simulink model "bitsel"  (Simulink 6.2)
settings: Solver=ode45  StartTime=0.0  StopTime=10.0  RelTol=1e-3
libraries: xbsIndex_r3 x74
settings Model: LastModifiedBy=mdexter
settings DebuggingCC: SolverPrmCheckMsg=warning

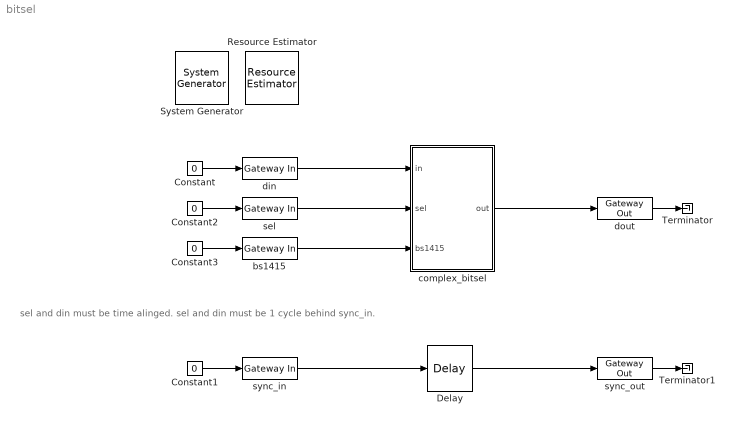
== system bitsel ==
  note: sel and din must be time alinged.
      | sel and din must be 1 cycle behind sync_in.
  " System Generator" : xbsIndex_r3/ System Generator  Tag=genX  xilinxfamily=Virtex2P  part=xc2vp40  speed=-6  package=ff1152  synthesis_tool=XST  directory=./bitsel_core  testbench=off  simulink_period=1  sysclk_period=100  incr_netlist=off  trim_vbits=Everywhere in SubSystem  dbl_ovrd=According to Block Masks  core_generation=According to Block Masks  run_coregen=off  deprecated_control=off  eval_field=0
      settings: AttributesFormatString=System\nGenerator
  Constant{,1..3} (4 alike) : Constant  Value=0
  Delay : xbsIndex_r3/Delay  latency=2  reg_retiming=off  explicit_period=off  period=1  en=off  accept_only_valid=off  init_zero=on  dbl_ovrd=off  show_param=off
      settings: xl_area=[1 1 0 1 0 0 0]
  Resource Estimator : xbsIndex_r3/Resource Estimator  Tag=resEstTag  xl_estimator_area=[342 135 0 641 52 0 0]  xl_use_estimator_area=off  simulink_period=1  mrp_directory=./bitsel_core
      settings: AttributesFormatString=Resource\nEstimator
  Terminator : Terminator
  Terminator1 : Terminator
  bs1415 : xbsIndex_r3/Gateway In  arith_type=Unsigned  n_bits=16  bin_pt=0  quantization=Truncate  overflow=Wrap  period=1  timing_constraint=None  locs_specified=off  LOCs={}  needs_fixed_name=off  dbl_ovrd=off  show_param=off
      settings: xl_area=[0 0 0 0 4 0 0]
  complex_bitsel : Subsystem
      settings: AttributesFormatString=latency = 2
  din : xbsIndex_r3/Gateway In  arith_type=Unsigned  n_bits=38  bin_pt=0  quantization=Truncate  overflow=Wrap  period=1  timing_constraint=None  locs_specified=off  LOCs={}  needs_fixed_name=off  dbl_ovrd=off  show_param=off
      settings: xl_area=[0 0 0 0 38 0 0]
  dout : xbsIndex_r3/Gateway Out  output_type=Double  nbits=8  bin_pt=6  arith_type=Boolean  quantization=Truncate  overflow=Wrap  hdl_port=on  timing_constraint=None  locs_specified=off  LOCs={}  needs_fixed_name=off  show_param=off
      settings: xl_area=[0 0 0 0 8 0 0]
  sel : xbsIndex_r3/Gateway In  arith_type=Unsigned  n_bits=4  bin_pt=0  quantization=Truncate  overflow=Wrap  period=1  timing_constraint=None  locs_specified=off  LOCs={}  needs_fixed_name=off  dbl_ovrd=off  show_param=off
      settings: xl_area=[0 0 0 0 4 0 0]
  sync_in : xbsIndex_r3/Gateway In  arith_type=Boolean  n_bits=36  bin_pt=0  quantization=Truncate  overflow=Wrap  period=1  timing_constraint=None  locs_specified=off  LOCs={}  needs_fixed_name=off  dbl_ovrd=off  show_param=off
      settings: xl_area=[0 0 0 0 1 0 0]
  sync_out : xbsIndex_r3/Gateway Out  output_type=Double  nbits=8  bin_pt=6  arith_type=Boolean  quantization=Truncate  overflow=Wrap  hdl_port=on  timing_constraint=None  locs_specified=off  LOCs={}  needs_fixed_name=off  show_param=off
      settings: xl_area=[0 0 0 0 1 0 0]
  wires:
  Constant/1 -> din/1
  Constant2/1 -> sel/1
  dout/1 -> Terminator/1
  Constant1/1 -> sync_in/1
  sync_out/1 -> Terminator1/1
  sync_in/1 -> Delay/1
  Delay/1 -> sync_out/1
  din/1 -> complex_bitsel/1(in)
  sel/1 -> complex_bitsel/2(sel)
  complex_bitsel/1(out) -> dout/1
  Constant3/1 -> bs1415/1
  bs1415/1 -> complex_bitsel/3(bs1415)

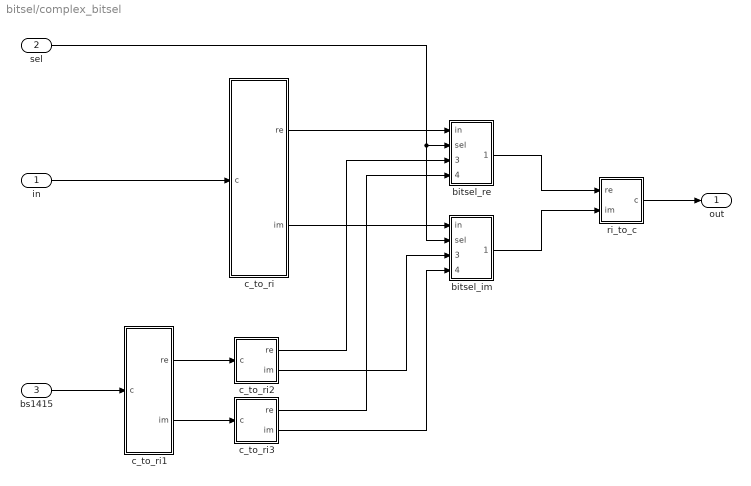
== system bitsel/complex_bitsel ==
  in : Inport  Port=1  LatchInput=off
  sel : Inport  Port=2  LatchInput=off
  bs1415 : Inport  Port=3  LatchInput=off
  bitsel_im : Subsystem
      settings: AttributesFormatString=latency = 2
  bitsel_re : Subsystem
      settings: AttributesFormatString=latency = 2
  c_to_ri : Subsystem  mask(Complex to Real-Imag){n_bits=19, bin_pt=0}
      mask prompts: n_bits "Bit Width"; bin_pt "Binary Point"
      mask help: Outputs real and imaginary components of a complex input.
      mask init:
      | c_to_ri_init(gcb,n_bits,bin_pt);
      settings: AttributesFormatString=19_0 r/i
      mask Help:
      | <pre>
      | Description::
      | 
      | Outputs real and imaginary components of a complex input.
      | Useful for simplifying interconnects.
      | See also: Real-Imag to Complex (ri_to_c)
      | 
      | Mask Parameters::
      | 
      | Bit Width (n_bits): Specifies the width of the real/imaginary components.
      | Assumed equal for both components.
      | 
      | Binary Point (bin_pt): Specifies the binary point location in the real/imaginary components.
      | Assumed equal for both components.
      | </pre>
  c_to_ri1 : Subsystem  mask(Complex to Real-Imag){n_bits=8, bin_pt=0}
      mask prompts: n_bits "Bit Width"; bin_pt "Binary Point"
      mask help: Outputs real and imaginary components of a complex input.
      mask init:
      | c_to_ri_init(gcb,n_bits,bin_pt);
      settings: AttributesFormatString=8_0 r/i
      mask Help:
      | <pre>
      | Description::
      | 
      | Outputs real and imaginary components of a complex input.
      | Useful for simplifying interconnects.
      | See also: Real-Imag to Complex (ri_to_c)
      | 
      | Mask Parameters::
      | 
      | Bit Width (n_bits): Specifies the width of the real/imaginary components.
      | Assumed equal for both components.
      | 
      | Binary Point (bin_pt): Specifies the binary point location in the real/imaginary components.
      | Assumed equal for both components.
      | </pre>
  c_to_ri2 : Subsystem  mask(Complex to Real-Imag){n_bits=4, bin_pt=0}
      mask prompts: n_bits "Bit Width"; bin_pt "Binary Point"
      mask help: Outputs real and imaginary components of a complex input.
      mask init:
      | c_to_ri_init(gcb,n_bits,bin_pt);
      settings: AttributesFormatString=4_0 r/i
      mask Help:
      | <pre>
      | Description::
      | 
      | Outputs real and imaginary components of a complex input.
      | Useful for simplifying interconnects.
      | See also: Real-Imag to Complex (ri_to_c)
      | 
      | Mask Parameters::
      | 
      | Bit Width (n_bits): Specifies the width of the real/imaginary components.
      | Assumed equal for both components.
      | 
      | Binary Point (bin_pt): Specifies the binary point location in the real/imaginary components.
      | Assumed equal for both components.
      | </pre>
  c_to_ri3 : Subsystem  mask(Complex to Real-Imag){n_bits=4, bin_pt=0}
      mask prompts: n_bits "Bit Width"; bin_pt "Binary Point"
      mask help: Outputs real and imaginary components of a complex input.
      mask init:
      | c_to_ri_init(gcb,n_bits,bin_pt);
      settings: AttributesFormatString=4_0 r/i
      mask Help:
      | <pre>
      | Description::
      | 
      | Outputs real and imaginary components of a complex input.
      | Useful for simplifying interconnects.
      | See also: Real-Imag to Complex (ri_to_c)
      | 
      | Mask Parameters::
      | 
      | Bit Width (n_bits): Specifies the width of the real/imaginary components.
      | Assumed equal for both components.
      | 
      | Binary Point (bin_pt): Specifies the binary point location in the real/imaginary components.
      | Assumed equal for both components.
      | </pre>
  ri_to_c : Subsystem  mask(Real-Imag to Complex){}
      mask help: Concatenates real and imaginary inputs into a complex output.
      mask init:
      | ri_to_c_init(gcb);
      mask Help:
      | <pre>
      | Description::
      | 
      | Concatenates a real and imaginary input into a complex output.
      | Useful for simplifying interconnects.
      | See also: Complex to Real-Imag (c_to_ri)
      | 
      | Mask Parameters::
      | 
      | (N/A)
      | </pre>
  out : Outport
  wires:
  in/1 -> c_to_ri/1(c)
  sel/1 -> bitsel_im/2(sel), bitsel_re/2(sel)
  c_to_ri/1(re) -> bitsel_re/1(in)
  c_to_ri/2(im) -> bitsel_im/1(in)
  bitsel_re/1(out) -> ri_to_c/1(re)
  ri_to_c/1(c) -> out/1
  bitsel_im/1(out) -> ri_to_c/2(im)
  c_to_ri1/1(re) -> c_to_ri2/1(c)
  c_to_ri1/2(im) -> c_to_ri3/1(c)
  c_to_ri2/1(re) -> bitsel_re/3(bs14)
  c_to_ri3/1(re) -> bitsel_re/4(bs15)
  c_to_ri2/2(im) -> bitsel_im/3(bs14)
  c_to_ri3/2(im) -> bitsel_im/4(bs15)
  bs1415/1 -> c_to_ri1/1(c)

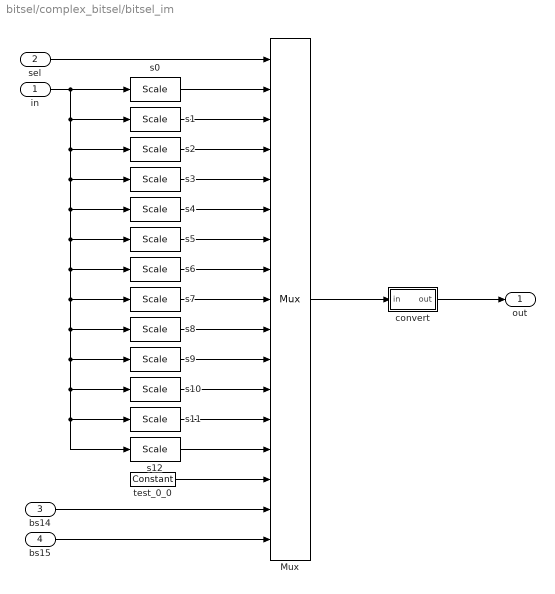
== system bitsel/complex_bitsel/bitsel_im ==
  in : Inport  Port=1  LatchInput=off
  sel : Inport  Port=2  LatchInput=off
  bs14 : Inport  Port=3  LatchInput=off
  bs15 : Inport  Port=4  LatchInput=off
  Mux : xbsIndex_r3/Mux  inputs=16  precision=Full  arith_type="Signed  (2's comp)"  n_bits=8  bin_pt=2  quantization=Truncate  overflow=Wrap  latency=1  explicit_period=off  period=1  en=off  dbl_ovrd=off  show_param=on  mux_type=off  use_rpm=on  gen_core=off
      settings: xl_area=[140 31 0 279 0 0 0]
  convert : Subsystem  mask(Convert (cast)){bin_pt_in=15, n_bits_out=4, bin_pt_out=0, quantization=Round  (unbiased: Even Values), overflow=Saturate, latency=1}
      mask prompts: bin_pt_in "Binary Point In"; n_bits_out "Bit Width Out"; bin_pt_out "Binary Point Out"
      mask help: Convert input value to the specified bit width and precision.
      mask init:
      | convert_init(gcb, ...
      |     bin_pt_in, ...
      |     n_bits_out,bin_pt_out, ...
      |     quantization,overflow,latency);
      settings: AttributesFormatString=|
      | N_15 ==> 4_0
      | round even, saturate
      | latency = 1
      mask Help:
      | <pre>
      | Description::
      | 
      | Outputs converted version of the input.
      | 
      | Mask Parameters::
      | 
      | Binary Point In (bin_pt_in): Specifies the binary point location in the input.
      | 
      | Bit Width Out (n_bits_out): Specifies the width of the output.
      | 
      | Binary Point Out (bin_pt_out): Specifies the binary point location in the output.
      | 
      | Quantization (quantization): Specifies quantization handling.
      | 
      | Overflow (overflow): Specifies overflow handling.
      | 
      | Latency (latency): Specifies the latency of the underlying adder block, which is the overall
      | latency of this block as well.
      | </pre>
      mask StyleString: edit,edit,edit,popup(Truncate|Round  (unbiased: +/- Inf)|Round  (unbiased: Even Values)|Round  (unbiased: Zero)|Round  (unbiased: Odd Values)|Round  (biased: Up)|Round  (biased: Down)),popup(Wrap|Saturate|Error),edit
  s0 : xbsIndex_r3/Scale  scale_factor=-15  explicit_period=off  period=1  dbl_ovrd=off
  s1 : xbsIndex_r3/Scale  scale_factor=-14  explicit_period=off  period=1  dbl_ovrd=off
  s10 : xbsIndex_r3/Scale  scale_factor=-5  explicit_period=off  period=1  dbl_ovrd=off
  s11 : xbsIndex_r3/Scale  scale_factor=-4  explicit_period=off  period=1  dbl_ovrd=off
  s12 : xbsIndex_r3/Scale  scale_factor=-3  explicit_period=off  period=1  dbl_ovrd=off
  s2 : xbsIndex_r3/Scale  scale_factor=-13  explicit_period=off  period=1  dbl_ovrd=off
  s3 : xbsIndex_r3/Scale  scale_factor=-12  explicit_period=off  period=1  dbl_ovrd=off
  s4 : xbsIndex_r3/Scale  scale_factor=-11  explicit_period=off  period=1  dbl_ovrd=off
  s5 : xbsIndex_r3/Scale  scale_factor=-10  explicit_period=off  period=1  dbl_ovrd=off
  s6 : xbsIndex_r3/Scale  scale_factor=-9  explicit_period=off  period=1  dbl_ovrd=off
  s7 : xbsIndex_r3/Scale  scale_factor=-8  explicit_period=off  period=1  dbl_ovrd=off
  s8 : xbsIndex_r3/Scale  scale_factor=-7  explicit_period=off  period=1  dbl_ovrd=off
  s9 : xbsIndex_r3/Scale  scale_factor=-6  explicit_period=off  period=1  dbl_ovrd=off
  test_0_0 : xbsIndex_r3/Constant  const=0  equ=P=C  arith_type="Signed  (2's comp)"  n_bits=4  bin_pt=0  opselect=C  inp2=PCIN>>17  opr=+  inp1=P  carry=CIN  iostate=0  explicit_period=on  period=1  dbl_ovrd=off
  out : Outport
  wires:
  in/1 -> s11/1, s12/1, s10/1, s9/1, s8/1, s7/1, s6/1, s5/1, s4/1, s3/1, s2/1, s1/1, s0/1
  s0/1 -> Mux/2
  s1/1 -> Mux/3
  s2/1 -> Mux/4
  s3/1 -> Mux/5
  s4/1 -> Mux/6
  s5/1 -> Mux/7
  s6/1 -> Mux/8
  s7/1 -> Mux/9
  s8/1 -> Mux/10
  s9/1 -> Mux/11
  s10/1 -> Mux/12
  s11/1 -> Mux/13
  s12/1 -> Mux/14
  test_0_0/1 -> Mux/15
  bs14/1 -> Mux/16
  bs15/1 -> Mux/17
  Mux/1 -> convert/1(in)
  sel/1 -> Mux/1
  convert/1(out) -> out/1

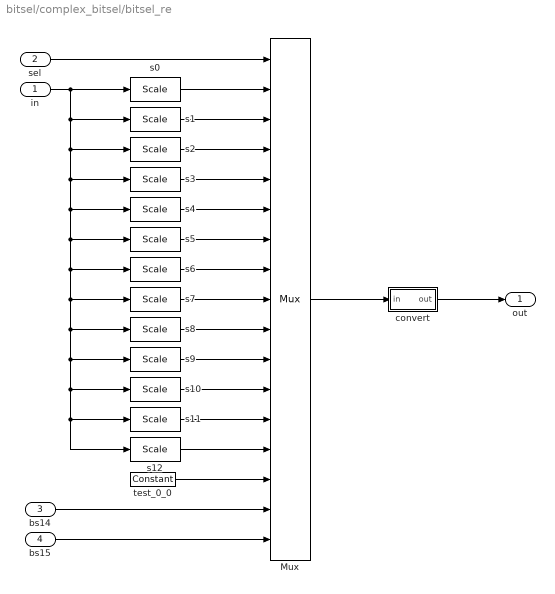
== system bitsel/complex_bitsel/bitsel_re ==
  in : Inport  Port=1  LatchInput=off
  sel : Inport  Port=2  LatchInput=off
  bs14 : Inport  Port=3  LatchInput=off
  bs15 : Inport  Port=4  LatchInput=off
  Mux : xbsIndex_r3/Mux  inputs=16  precision=Full  arith_type="Signed  (2's comp)"  n_bits=8  bin_pt=2  quantization=Truncate  overflow=Wrap  latency=1  explicit_period=off  period=1  en=off  dbl_ovrd=off  show_param=on  mux_type=off  use_rpm=on  gen_core=off
      settings: xl_area=[140 31 0 279 0 0 0]
  convert : Subsystem  mask(Convert (cast)){bin_pt_in=15, n_bits_out=4, bin_pt_out=0, quantization=Round  (unbiased: Even Values), overflow=Saturate, latency=1}
      mask prompts: bin_pt_in "Binary Point In"; n_bits_out "Bit Width Out"; bin_pt_out "Binary Point Out"
      mask help: Convert input value to the specified bit width and precision.
      mask init:
      | convert_init(gcb, ...
      |     bin_pt_in, ...
      |     n_bits_out,bin_pt_out, ...
      |     quantization,overflow,latency);
      settings: AttributesFormatString=|
      | N_15 ==> 4_0
      | round even, saturate
      | latency = 1
      mask Help:
      | <pre>
      | Description::
      | 
      | Outputs converted version of the input.
      | 
      | Mask Parameters::
      | 
      | Binary Point In (bin_pt_in): Specifies the binary point location in the input.
      | 
      | Bit Width Out (n_bits_out): Specifies the width of the output.
      | 
      | Binary Point Out (bin_pt_out): Specifies the binary point location in the output.
      | 
      | Quantization (quantization): Specifies quantization handling.
      | 
      | Overflow (overflow): Specifies overflow handling.
      | 
      | Latency (latency): Specifies the latency of the underlying adder block, which is the overall
      | latency of this block as well.
      | </pre>
      mask StyleString: edit,edit,edit,popup(Truncate|Round  (unbiased: +/- Inf)|Round  (unbiased: Even Values)|Round  (unbiased: Zero)|Round  (unbiased: Odd Values)|Round  (biased: Up)|Round  (biased: Down)),popup(Wrap|Saturate|Error),edit
  s0 : xbsIndex_r3/Scale  scale_factor=-15  explicit_period=off  period=1  dbl_ovrd=off
  s1 : xbsIndex_r3/Scale  scale_factor=-14  explicit_period=off  period=1  dbl_ovrd=off
  s10 : xbsIndex_r3/Scale  scale_factor=-5  explicit_period=off  period=1  dbl_ovrd=off
  s11 : xbsIndex_r3/Scale  scale_factor=-4  explicit_period=off  period=1  dbl_ovrd=off
  s12 : xbsIndex_r3/Scale  scale_factor=-3  explicit_period=off  period=1  dbl_ovrd=off
  s2 : xbsIndex_r3/Scale  scale_factor=-13  explicit_period=off  period=1  dbl_ovrd=off
  s3 : xbsIndex_r3/Scale  scale_factor=-12  explicit_period=off  period=1  dbl_ovrd=off
  s4 : xbsIndex_r3/Scale  scale_factor=-11  explicit_period=off  period=1  dbl_ovrd=off
  s5 : xbsIndex_r3/Scale  scale_factor=-10  explicit_period=off  period=1  dbl_ovrd=off
  s6 : xbsIndex_r3/Scale  scale_factor=-9  explicit_period=off  period=1  dbl_ovrd=off
  s7 : xbsIndex_r3/Scale  scale_factor=-8  explicit_period=off  period=1  dbl_ovrd=off
  s8 : xbsIndex_r3/Scale  scale_factor=-7  explicit_period=off  period=1  dbl_ovrd=off
  s9 : xbsIndex_r3/Scale  scale_factor=-6  explicit_period=off  period=1  dbl_ovrd=off
  test_0_0 : xbsIndex_r3/Constant  const=0  equ=P=C  arith_type="Signed  (2's comp)"  n_bits=4  bin_pt=0  opselect=C  inp2=PCIN>>17  opr=+  inp1=P  carry=CIN  iostate=0  explicit_period=on  period=1  dbl_ovrd=off
  out : Outport
  wires:
  in/1 -> s11/1, s12/1, s10/1, s9/1, s8/1, s7/1, s6/1, s5/1, s4/1, s3/1, s2/1, s1/1, s0/1
  s0/1 -> Mux/2
  s1/1 -> Mux/3
  s2/1 -> Mux/4
  s3/1 -> Mux/5
  s4/1 -> Mux/6
  s5/1 -> Mux/7
  s6/1 -> Mux/8
  s7/1 -> Mux/9
  s8/1 -> Mux/10
  s9/1 -> Mux/11
  s10/1 -> Mux/12
  s11/1 -> Mux/13
  s12/1 -> Mux/14
  test_0_0/1 -> Mux/15
  bs14/1 -> Mux/16
  bs15/1 -> Mux/17
  Mux/1 -> convert/1(in)
  sel/1 -> Mux/1
  convert/1(out) -> out/1

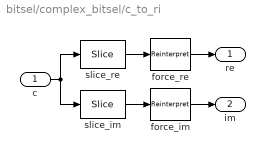
== system bitsel/complex_bitsel/c_to_ri ==
  c : Inport  Port=1  LatchInput=off
  force_im : xbsIndex_r3/Reinterpret  force_arith_type=on  arith_type="Signed  (2's comp)"  force_bin_pt=on  bin_pt=0  force_valid=on
  force_re : xbsIndex_r3/Reinterpret  force_arith_type=on  arith_type="Signed  (2's comp)"  force_bin_pt=on  bin_pt=0  force_valid=on
  slice_im : xbsIndex_r3/Slice  mode=Lower Bit Location + Width  nbits=19  bit1=0  base1=MSB of Input  bit0=0  base0=LSB of Input  boolean_output=off  explicit_period=off  period=1  dbl_ovrd=off
  slice_re : xbsIndex_r3/Slice  mode=Upper Bit Location + Width  nbits=19  bit1=0  base1=MSB of Input  bit0=0  base0=LSB of Input  boolean_output=off  explicit_period=off  period=1  dbl_ovrd=off
  re : Outport
  im : Outport  Port=2
  wires:
  slice_re/1 -> force_re/1
  slice_im/1 -> force_im/1
  force_re/1 -> re/1
  force_im/1 -> im/1
  c/1 -> slice_re/1, slice_im/1

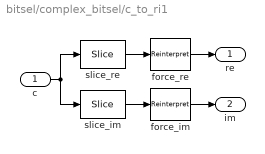
== system bitsel/complex_bitsel/c_to_ri1 ==
  c : Inport  Port=1  LatchInput=off
  force_im : xbsIndex_r3/Reinterpret  force_arith_type=on  arith_type="Signed  (2's comp)"  force_bin_pt=on  bin_pt=0  force_valid=on
  force_re : xbsIndex_r3/Reinterpret  force_arith_type=on  arith_type="Signed  (2's comp)"  force_bin_pt=on  bin_pt=0  force_valid=on
  slice_im : xbsIndex_r3/Slice  mode=Lower Bit Location + Width  nbits=8  bit1=0  base1=MSB of Input  bit0=0  base0=LSB of Input  boolean_output=off  explicit_period=off  period=1  dbl_ovrd=off
  slice_re : xbsIndex_r3/Slice  mode=Upper Bit Location + Width  nbits=8  bit1=0  base1=MSB of Input  bit0=0  base0=LSB of Input  boolean_output=off  explicit_period=off  period=1  dbl_ovrd=off
  re : Outport
  im : Outport  Port=2
  wires:
  slice_re/1 -> force_re/1
  slice_im/1 -> force_im/1
  force_re/1 -> re/1
  force_im/1 -> im/1
  c/1 -> slice_re/1, slice_im/1

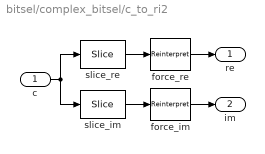
== system bitsel/complex_bitsel/c_to_ri2 ==
  c : Inport  Port=1  LatchInput=off
  force_im : xbsIndex_r3/Reinterpret  force_arith_type=on  arith_type="Signed  (2's comp)"  force_bin_pt=on  bin_pt=0  force_valid=on
  force_re : xbsIndex_r3/Reinterpret  force_arith_type=on  arith_type="Signed  (2's comp)"  force_bin_pt=on  bin_pt=0  force_valid=on
  slice_im : xbsIndex_r3/Slice  mode=Lower Bit Location + Width  nbits=4  bit1=0  base1=MSB of Input  bit0=0  base0=LSB of Input  boolean_output=off  explicit_period=off  period=1  dbl_ovrd=off
  slice_re : xbsIndex_r3/Slice  mode=Upper Bit Location + Width  nbits=4  bit1=0  base1=MSB of Input  bit0=0  base0=LSB of Input  boolean_output=off  explicit_period=off  period=1  dbl_ovrd=off
  re : Outport
  im : Outport  Port=2
  wires:
  slice_re/1 -> force_re/1
  slice_im/1 -> force_im/1
  force_re/1 -> re/1
  force_im/1 -> im/1
  c/1 -> slice_re/1, slice_im/1

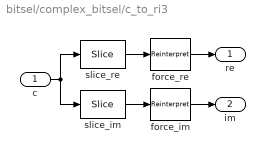
== system bitsel/complex_bitsel/c_to_ri3 ==
  c : Inport  Port=1  LatchInput=off
  force_im : xbsIndex_r3/Reinterpret  force_arith_type=on  arith_type="Signed  (2's comp)"  force_bin_pt=on  bin_pt=0  force_valid=on
  force_re : xbsIndex_r3/Reinterpret  force_arith_type=on  arith_type="Signed  (2's comp)"  force_bin_pt=on  bin_pt=0  force_valid=on
  slice_im : xbsIndex_r3/Slice  mode=Lower Bit Location + Width  nbits=4  bit1=0  base1=MSB of Input  bit0=0  base0=LSB of Input  boolean_output=off  explicit_period=off  period=1  dbl_ovrd=off
  slice_re : xbsIndex_r3/Slice  mode=Upper Bit Location + Width  nbits=4  bit1=0  base1=MSB of Input  bit0=0  base0=LSB of Input  boolean_output=off  explicit_period=off  period=1  dbl_ovrd=off
  re : Outport
  im : Outport  Port=2
  wires:
  slice_re/1 -> force_re/1
  slice_im/1 -> force_im/1
  force_re/1 -> re/1
  force_im/1 -> im/1
  c/1 -> slice_re/1, slice_im/1

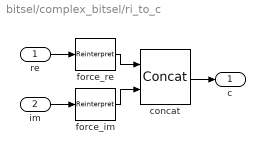
== system bitsel/complex_bitsel/ri_to_c ==
  re : Inport  Port=1  LatchInput=off
  im : Inport  Port=2  LatchInput=off
  concat : xbsIndex_r3/Concat  num_inputs=2  explicit_period=off  period=1  dbl_ovrd=off
  force_im : xbsIndex_r3/Reinterpret  force_arith_type=on  arith_type=Unsigned  force_bin_pt=on  bin_pt=0  force_valid=on
  force_re : xbsIndex_r3/Reinterpret  force_arith_type=on  arith_type=Unsigned  force_bin_pt=on  bin_pt=0  force_valid=on
  c : Outport
  wires:
  force_re/1 -> concat/1
  force_im/1 -> concat/2
  re/1 -> force_re/1
  concat/1 -> c/1
  im/1 -> force_im/1

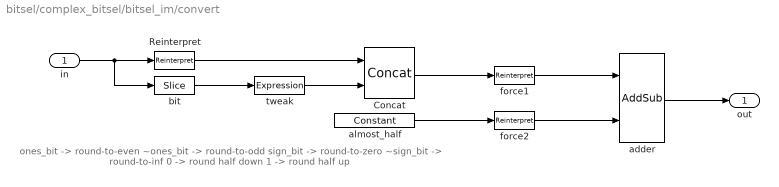
== system bitsel/complex_bitsel/bitsel_im/convert ==
  note: ones_bit -> round-to-even
      | ~ones_bit -> round-to-odd
      | sign_bit -> round-to-zero
      | ~sign_bit -> round-to-inf
      | 0 -> round half down
      | 1 -> round half up
  in : Inport  Port=1  LatchInput=off
  Concat : xbsIndex_r3/Concat  num_inputs=2  explicit_period=off  period=1  dbl_ovrd=off
  Reinterpret : xbsIndex_r3/Reinterpret  force_arith_type=on  arith_type=Unsigned  force_bin_pt=on  bin_pt=0  force_valid=on
  adder : xbsIndex_r3/AddSub  mode=Addition  precision=User Defined  arith_type="Signed  (2's comp)"  n_bits=4  bin_pt=0  quantization=Truncate  overflow=Saturate  latency=1  explicit_period=off  period=1  use_carryin=off  use_carryout=off  en=off  dbl_ovrd=off  show_param=on  use_core=on  pipeline=on  use_rpm=on  gen_core=off
      settings: xl_area=[21 17 0 41 0 0 0]
  almost_half : xbsIndex_r3/Constant  const=32767  equ=P=C  arith_type=Unsigned  n_bits=16  bin_pt=0  opselect=C  inp2=PCIN>>17  opr=+  inp1=P  carry=CIN  iostate=0  explicit_period=on  period=1  dbl_ovrd=off
  bit : xbsIndex_r3/Slice  mode=Lower Bit Location + Width  nbits=1  bit1=0  base1=MSB of Input  bit0=15  base0=LSB of Input  boolean_output=off  explicit_period=off  period=1  dbl_ovrd=off
  force1 : xbsIndex_r3/Reinterpret  force_arith_type=on  arith_type="Signed  (2's comp)"  force_bin_pt=on  bin_pt=16  force_valid=on
  force2 : xbsIndex_r3/Reinterpret  force_arith_type=off  arith_type="Signed  (2's comp)"  force_bin_pt=on  bin_pt=16  force_valid=on
  tweak : xbsIndex_r3/Expression  expression=a  precision=Full  arith_type=Unsigned  n_bits=8  bin_pt=2  align_bp=off  latency=0  explicit_period=off  period=1  en=off  dbl_ovrd=off  show_param=on
      settings: xl_area=[0, 0, 0, 0, 0, 0, 0]
  out : Outport
  wires:
  bit/1 -> tweak/1
  almost_half/1 -> force2/1
  in/1 -> Reinterpret/1, bit/1
  Concat/1 -> force1/1
  Reinterpret/1 -> Concat/1
  tweak/1 -> Concat/2
  force1/1 -> adder/1
  force2/1 -> adder/2
  adder/1 -> out/1

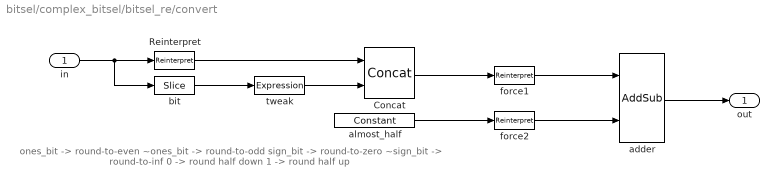
== system bitsel/complex_bitsel/bitsel_re/convert ==
  note: ones_bit -> round-to-even
      | ~ones_bit -> round-to-odd
      | sign_bit -> round-to-zero
      | ~sign_bit -> round-to-inf
      | 0 -> round half down
      | 1 -> round half up
  in : Inport  Port=1  LatchInput=off
  Concat : xbsIndex_r3/Concat  num_inputs=2  explicit_period=off  period=1  dbl_ovrd=off
  Reinterpret : xbsIndex_r3/Reinterpret  force_arith_type=on  arith_type=Unsigned  force_bin_pt=on  bin_pt=0  force_valid=on
  adder : xbsIndex_r3/AddSub  mode=Addition  precision=User Defined  arith_type="Signed  (2's comp)"  n_bits=4  bin_pt=0  quantization=Truncate  overflow=Saturate  latency=1  explicit_period=off  period=1  use_carryin=off  use_carryout=off  en=off  dbl_ovrd=off  show_param=on  use_core=on  pipeline=on  use_rpm=on  gen_core=off
      settings: xl_area=[21 17 0 41 0 0 0]
  almost_half : xbsIndex_r3/Constant  const=32767  equ=P=C  arith_type=Unsigned  n_bits=16  bin_pt=0  opselect=C  inp2=PCIN>>17  opr=+  inp1=P  carry=CIN  iostate=0  explicit_period=on  period=1  dbl_ovrd=off
  bit : xbsIndex_r3/Slice  mode=Lower Bit Location + Width  nbits=1  bit1=0  base1=MSB of Input  bit0=15  base0=LSB of Input  boolean_output=off  explicit_period=off  period=1  dbl_ovrd=off
  force1 : xbsIndex_r3/Reinterpret  force_arith_type=on  arith_type="Signed  (2's comp)"  force_bin_pt=on  bin_pt=16  force_valid=on
  force2 : xbsIndex_r3/Reinterpret  force_arith_type=off  arith_type="Signed  (2's comp)"  force_bin_pt=on  bin_pt=16  force_valid=on
  tweak : xbsIndex_r3/Expression  expression=a  precision=Full  arith_type=Unsigned  n_bits=8  bin_pt=2  align_bp=off  latency=0  explicit_period=off  period=1  en=off  dbl_ovrd=off  show_param=on
      settings: xl_area=[0, 0, 0, 0, 0, 0, 0]
  out : Outport
  wires:
  bit/1 -> tweak/1
  almost_half/1 -> force2/1
  in/1 -> Reinterpret/1, bit/1
  Concat/1 -> force1/1
  Reinterpret/1 -> Concat/1
  tweak/1 -> Concat/2
  force1/1 -> adder/1
  force2/1 -> adder/2
  adder/1 -> out/1
